simulink model "chap5_2sim"  (Simulink 8.1)
settings: Solver=ode45  StartTime=0.0  StopTime=20  FixedStep=0.001  RelTol=1e-3
settings Model: Creator=ljk  LastModifiedBy=liujk  ExtModeTrigMode=oneshot  ExtModeArmWhenConnect=off
settings DataIOCC: LimitDataPoints=off  SignalLoggingName=sigsOut
settings OptimizationCC: BooleanDataType=off
settings DebuggingCC: SaveWithParameterizedLinksMsg=none  SignalResolutionControl=TryResolveAllWithWarning  SolverPrmCheckMsg=none  MultiTaskDSMMsg=warning  MultiTaskCondExecSysMsg=none  StrictBusMsg=None
settings HardwareCC: TargetUnknown=on
settings RTWCC: IncludeERTFirstTime=on

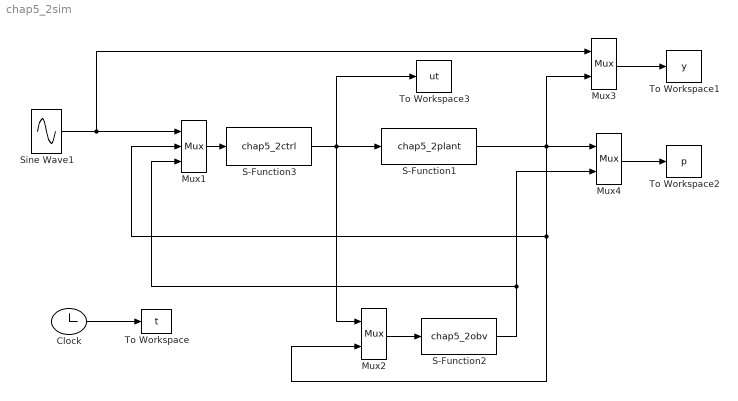
== system chap5_2sim ==
  Clock : Clock
  Mux1 : Mux  Inputs=3
  Mux2 : Mux  Inputs=2
  Mux3 : Mux  Inputs=2
  Mux4 : Mux  Inputs=2
  S-Function1 : S-Function  FunctionName=chap5_2plant  EnableBusSupport=off
  S-Function2 : S-Function  FunctionName=chap5_2obv  EnableBusSupport=off
  S-Function3 : S-Function  FunctionName=chap5_2ctrl  EnableBusSupport=off
  Sine Wave1 : Sin  SampleTime=0
  To Workspace : ToWorkspace  VariableName=t  SampleTime=-1
  To Workspace1 : ToWorkspace  VariableName=y  SampleTime=-1
  To Workspace2 : ToWorkspace  VariableName=p  SampleTime=-1
  To Workspace3 : ToWorkspace  VariableName=ut  SampleTime=-1
  wires:
  S-Function1/1 -> Mux4/1, Mux2/2, Mux1/2, Mux3/2
  Clock/1 -> To Workspace/1
  Mux4/1 -> To Workspace2/1
  Sine Wave1/1 -> Mux3/1, Mux1/1
  S-Function2/1 -> Mux4/2, Mux1/3
  Mux2/1 -> S-Function2/1
  Mux3/1 -> To Workspace1/1
  S-Function3/1 -> S-Function1/1, To Workspace3/1, Mux2/1
  Mux1/1 -> S-Function3/1
